simulink model "PulseSessionMaster_SL_sim"  (R2016a)
settings: Solver=FixedStepDiscrete  StartTime=0.0  StopTime=inf  FixedStep=sCoreParams.core.stepPeriod  RelTol=1e-3
PreLoadFcn:
  | sCoreParams = InitCoreParams;
settings Model: ExplicitPartitioning=on  Creator=User  LastModifiedBy=rzelmann
settings SolverCC: EnableConcurrentExecution=on
settings DataIOCC: SaveFormat=Array  SaveOutput=off  SignalLogging=off  DSMLogging=off  SaveTime=off
settings OptimizationCC: BlockReduction=off  DefaultParameterBehavior=Inlined  InlineInvariantSignals=on  EnhancedBackFolding=on
settings DebuggingCC: UnderspecifiedInitializationDetection=Classic  MergeDetectMultiDrivingBlocksExec=none  SolverPrmCheckMsg=warning  StateNameClashWarn=warning
settings HardwareCC: ProdBitPerPointer=32  ProdLargestAtomicFloat=None  ProdWordSize=32  ProdLongLongMode=on  ProdHWDeviceType=Generic->32-bit x86 compatible
settings ModelReferenceCC: UpdateModelReferenceTargets=Force  EnableParallelModelReferenceBuilds=on  ParallelModelReferenceMATLABWorkerInit=Load Top Model  ModelReferenceNumInstancesAllowed=Single  ModelReferenceMinAlgLoopOccurrences=on  PropagateSignalLabelsOutOfModel=off
settings RTWCC: SystemTargetFile=slrt.tlc  TemplateMakefile=slrt_default_tmf  Description=Simulink Real-Time  RTWCompilerOptimization=on
settings SimulinkRealTimeCC: GeneratePreprocessorConditionals=Disable all
settings ConfigComp: CovModelRefEnable=Off  CovSFcnEnable=off

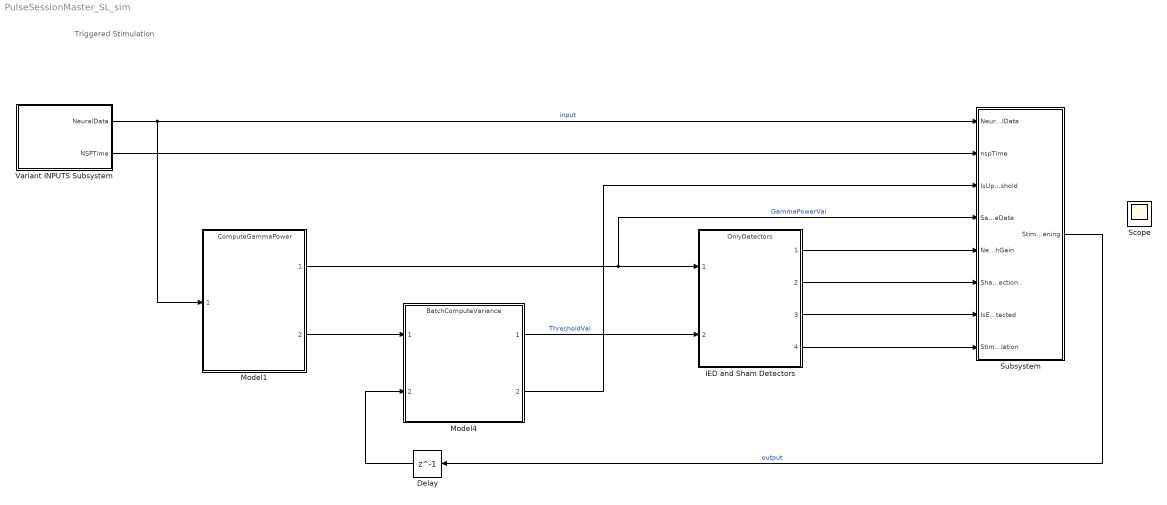
== system PulseSessionMaster_SL_sim ==
  note: Triggered Stimulation
  Delay : Delay  DelayLength=1  InitialCondition=0
  IED and Sham Detectors : ModelReference  ModelNameDialog=OnlyDetectors  SimulationMode=Normal  ModelReferenceVersion=1.219
  Model1 : ModelReference  ModelNameDialog=ComputeGammaPower.slx  SimulationMode=Normal  ModelReferenceVersion=1.119
  Model4 : ModelReference  ModelNameDialog=BatchComputeVariance.slx  SimulationMode=Normal  ModelReferenceVersion=1.112
  Scope : Scope
      settings: Floating=on
  Subsystem : Subsystem
  Variant INPUTS Subsystem : Subsystem  Description=|  Variant=on
      | Variant to use random generator during simulations 
      | or real Network inputs (from NSP) during Deployment with Target PC
  wires:
  Variant INPUTS Subsystem/1(NeuralData) -> Model1/1, Subsystem/1(NeuralData)  "input"
  Model4/1 -> IED and Sham Detectors/2  "ThresholdVal"
  Model1/1 -> Subsystem/4(SampleData), IED and Sham Detectors/1  "GammaPowerVal"
  Subsystem/1(StimHappening) -> Delay/1  "output"
  Model1/2 -> Model4/1
  IED and Sham Detectors/2 -> Subsystem/6(ShamDetection)
  IED and Sham Detectors/3 -> Subsystem/7(IsEventDetected)
  IED and Sham Detectors/4 -> Subsystem/8(Stimulation)
  IED and Sham Detectors/1 -> Subsystem/5(NewDataStdwithGain)
  Delay/1 -> Model4/2
  Variant INPUTS Subsystem/2(NSPTime) -> Subsystem/2(nspTime)
  Model4/2 -> Subsystem/3(IsUpdatingThreshold)

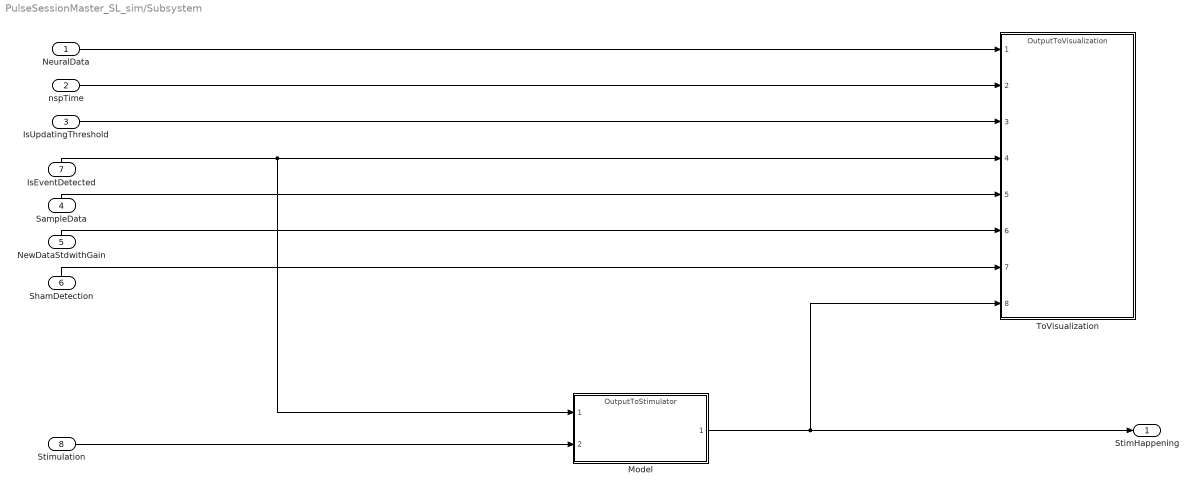
== system PulseSessionMaster_SL_sim/Subsystem ==
  NeuralData : Inport
  nspTime : Inport  Port=2
  IsUpdatingThreshold : Inport  Port=3
  SampleData : Inport  Port=4
  NewDataStdwithGain : Inport  Port=5
  ShamDetection : Inport  Port=6
  IsEventDetected : Inport  Port=7
  Stimulation : Inport  Port=8
  Model : ModelReference  ModelNameDialog=OutputToStimulator  SimulationMode=Normal  ModelReferenceVersion=1.6
  ToVisualization : ModelReference  ModelNameDialog=OutputToVisualization  SimulationMode=Normal  ModelReferenceVersion=1.27
  StimHappening : Outport
  wires:
  IsEventDetected/1 -> ToVisualization/4, Model/1
  IsUpdatingThreshold/1 -> ToVisualization/3
  nspTime/1 -> ToVisualization/2
  ShamDetection/1 -> ToVisualization/7
  Model/1 -> ToVisualization/8, StimHappening/1
  Stimulation/1 -> Model/2
  SampleData/1 -> ToVisualization/5
  NewDataStdwithGain/1 -> ToVisualization/6
  NeuralData/1 -> ToVisualization/1

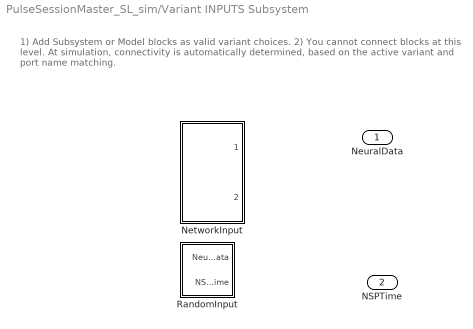
== system PulseSessionMaster_SL_sim/Variant INPUTS Subsystem ==
  note: 1) Add Subsystem or Model blocks as valid variant choices.
      | 2) You cannot connect blocks at this level. At simulation, connectivity is automatically
      | determined, based on the active variant and port name matching.
  NetworkInput : ModelReference  ModelNameDialog=NetworkReceive  VariantControl=(default)  ModelReferenceVersion=1.156
  RandomInput : Subsystem  VariantControl=simulation == 1
  NeuralData : Outport
  NSPTime : Outport  Port=2

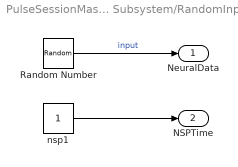
== system PulseSessionMaster_SL_sim/Variant INPUTS Subsystem/RandomInput ==
  Random Number : RandomNumber  Mean=zeros(2,200)  Variance=10  SampleTime=0.001
  nsp1 : Constant
  NeuralData : Outport
  NSPTime : Outport  Port=2
  wires:
  nsp1/1 -> NSPTime/1
  Random Number/1 -> NeuralData/1  "input"
